simulink model "DMC_simulink_trial_1_MIMO"  (R2015a)
settings: Solver=ode45  StartTime=0.0  StopTime=900  RelTol=1e-3
values from neighbouring files (symbols this model uses):
  Fac = (inv(G'*G+lambda*eye(2*(M+1))))*(G')    [DMC_MIMO_DATA_Gen.m]    (also in DMC_SISO_DATA_Gen.m = (inv(G'*G+lambda*eye(M+1)))*(G'))
  temp_f = [temp_f_11 temp_f_12;temp_f_21 temp_f_22]    [DMC_MIMO_DATA_Gen.m]    (also in DMC_SISO_DATA_Gen.m = temp_g1 - temp_g2)
settings Model: Creator=Ronak  LastModifiedBy=Ronak

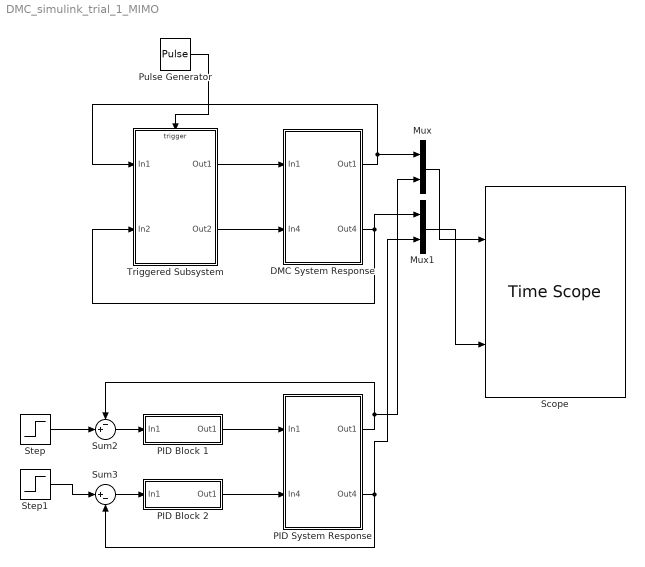
== system DMC_simulink_trial_1_MIMO ==
  DMC System Response : Subsystem
  Mux : Mux  Inputs=2
  Mux1 : Mux  Inputs=2
  PID Block 1 : Subsystem
  PID Block 2 : Subsystem
  PID System Response : Subsystem
  Pulse Generator : DiscretePulseGenerator  PulseType=Time based  Period=0.1  PulseWidth=5
  Scope : TimeScope  NumInputPorts=2
  Step : Step  SampleTime=0
  Step1 : Step  SampleTime=0
  Sum2 : Sum  Inputs=-+|
  Sum3 : Sum  Inputs=|+-
  Triggered Subsystem : Subsystem  TreatAsAtomicUnit=on
  wires:
  DMC System Response/1(Out1) -> Mux/1, Triggered Subsystem/1(In1)
  DMC System Response/2(Out4) -> Triggered Subsystem/2(In2), Mux1/1
  Pulse Generator/1 -> Triggered Subsystem/Trigger
  Triggered Subsystem/1(Out1) -> DMC System Response/1(In1)
  Triggered Subsystem/2(Out2) -> DMC System Response/2(In4)
  Mux/1 -> Scope/1
  Mux1/1 -> Scope/2
  PID Block 1/1(Out1) -> PID System Response/1(In1)
  PID Block 2/1(Out1) -> PID System Response/2(In4)
  Sum2/1 -> PID Block 1/1(In1)
  Sum3/1 -> PID Block 2/1(In1)
  Step/1 -> Sum2/2
  Step1/1 -> Sum3/1
  PID System Response/1(Out1) -> Mux/2, Sum2/1
  PID System Response/2(Out4) -> Sum3/2, Mux1/2

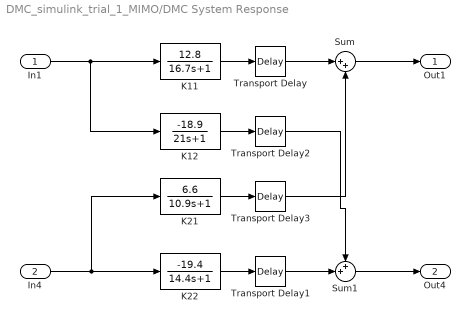
== system DMC_simulink_trial_1_MIMO/DMC System Response ==
  In1 : Inport
  In4 : Inport  Port=2
  K11 : TransferFcn  Numerator=[12.8]  Denominator=[16.7 1]
  K12 : TransferFcn  Numerator=[-18.9]  Denominator=[21 1]
  K21 : TransferFcn  Numerator=[6.6]  Denominator=[10.9 1]
  K22 : TransferFcn  Numerator=[-19.4]  Denominator=[14.4 1]
  Sum : Sum  Inputs=|++
  Sum1 : Sum  Inputs=++|
  Transport Delay : TransportDelay
  Transport Delay1 : TransportDelay  DelayTime=3
  Transport Delay2 : TransportDelay  DelayTime=3
  Transport Delay3 : TransportDelay  DelayTime=7
  Out1 : Outport
  Out4 : Outport  Port=2
  wires:
  In4/1 -> K21/1, K22/1
  K22/1 -> Transport Delay1/1
  In1/1 -> K12/1, K11/1
  Transport Delay1/1 -> Sum1/2
  K21/1 -> Transport Delay3/1
  K11/1 -> Transport Delay/1
  K12/1 -> Transport Delay2/1
  Sum1/1 -> Out4/1
  Sum/1 -> Out1/1
  Transport Delay/1 -> Sum/1
  Transport Delay2/1 -> Sum1/1
  Transport Delay3/1 -> Sum/2

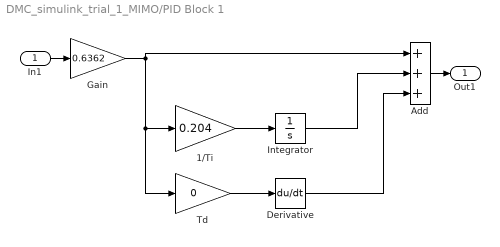
== system DMC_simulink_trial_1_MIMO/PID Block 1 ==
  In1 : Inport
  1/Ti : Gain  Gain=0.204
  Add : Sum  Inputs=+++
  Derivative : Derivative
  Gain : Gain  Gain=0.6362
  Integrator : Integrator
  Td : Gain  Gain=0
  Out1 : Outport
  wires:
  In1/1 -> Gain/1
  Add/1 -> Out1/1
  Gain/1 -> Add/1, Td/1, 1/Ti/1
  Integrator/1 -> Add/2
  Derivative/1 -> Add/3
  1/Ti/1 -> Integrator/1
  Td/1 -> Derivative/1

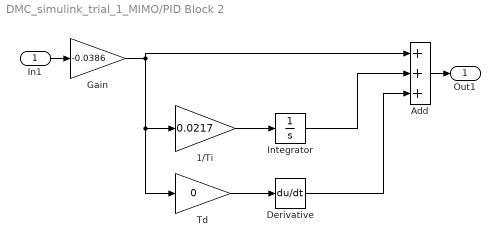
== system DMC_simulink_trial_1_MIMO/PID Block 2 ==
  In1 : Inport
  1/Ti : Gain  Gain=0.0217
  Add : Sum  Inputs=+++
  Derivative : Derivative
  Gain : Gain  Gain=-0.0386
  Integrator : Integrator
  Td : Gain  Gain=0
  Out1 : Outport
  wires:
  In1/1 -> Gain/1
  Add/1 -> Out1/1
  Gain/1 -> Add/1, Td/1, 1/Ti/1
  Integrator/1 -> Add/2
  Derivative/1 -> Add/3
  1/Ti/1 -> Integrator/1
  Td/1 -> Derivative/1

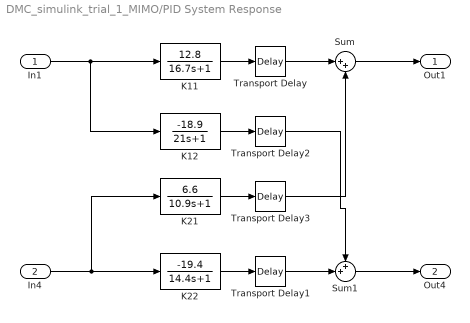
== system DMC_simulink_trial_1_MIMO/PID System Response ==
  In1 : Inport
  In4 : Inport  Port=2
  K11 : TransferFcn  Numerator=[12.8]  Denominator=[16.7 1]
  K12 : TransferFcn  Numerator=[-18.9]  Denominator=[21 1]
  K21 : TransferFcn  Numerator=[6.6]  Denominator=[10.9 1]
  K22 : TransferFcn  Numerator=[-19.4]  Denominator=[14.4 1]
  Sum : Sum  Inputs=|++
  Sum1 : Sum  Inputs=++|
  Transport Delay : TransportDelay
  Transport Delay1 : TransportDelay  DelayTime=3
  Transport Delay2 : TransportDelay  DelayTime=3
  Transport Delay3 : TransportDelay  DelayTime=7
  Out1 : Outport
  Out4 : Outport  Port=2
  wires:
  Transport Delay3/1 -> Sum/2
  Transport Delay2/1 -> Sum1/1
  Transport Delay/1 -> Sum/1
  Sum/1 -> Out1/1
  Sum1/1 -> Out4/1
  K12/1 -> Transport Delay2/1
  K11/1 -> Transport Delay/1
  K21/1 -> Transport Delay3/1
  Transport Delay1/1 -> Sum1/2
  In1/1 -> K11/1, K12/1
  K22/1 -> Transport Delay1/1
  In4/1 -> K22/1, K21/1

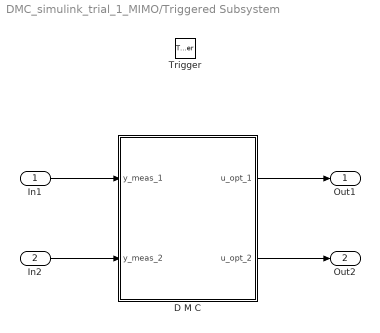
== system DMC_simulink_trial_1_MIMO/Triggered Subsystem ==
  In1 : Inport
  In2 : Inport  Port=2
  Trigger : TriggerPort
  D M C : MATLAB Function  TreatAsAtomicUnit=on
  Out1 : Outport
  Out2 : Outport  Port=2
  wires:
  In1/1 -> D M C/1(y_meas_1)
  D M C/1(u_opt_1) -> Out1/1
  D M C/2(u_opt_2) -> Out2/1
  In2/1 -> D M C/2(y_meas_2)

== matlab function DMC_simulink_trial_1_MIMO/Triggered Subsystem/D M C ==
  data: y_meas_1 input; y_meas_2 input; temp_f parameter; Fac parameter; u_opt_1 output; u_opt_2 output
function [u_opt_1,u_opt_2]    = fcn(y_meas_1,y_meas_2,temp_f,Fac)
%#codegen
coder.extrinsic('evalin', 'assignin')
r1 = y_meas_1;
r2 = y_meas_2;
y_sp_1 = 1;
y_sp_2 = 1;
alpha = 0.9;
u = zeros(2000,1);  % 2Nx1; past moves
u = evalin('base','u'); % Read value from workspace
u_old_1 = 0;
u_old_2 = 0;
u_old_1 = evalin('base','u_old_1'); 
u_old_2 = evalin('base','u_old_2'); 
ref_1 = zeros(1,900);       % 1,P
ref_2 = zeros(1,900);
for i =1:900    %1:P
    r1 = alpha*r1 + (1-alpha)*y_sp_1;
    r2 = alpha*r2 + (1-alpha)*y_sp_2;
    ref_1(i) = r1;
    ref_2(i) = r2;
end
ref = [ref_1';ref_2'];
f_1 = y_meas_1*ones(900,1);
f_2 = y_meas_2*ones(900,1);
y_meas = [f_1;f_2];
f = y_meas + temp_f*u; % Free Response
u_temp = Fac*(ref-f);
u_opt_1 = u_old_1 + u_temp(1);
u_opt_2 = u_old_2 + u_temp(601);
u = [u_temp(1);u(1:999);u_temp(601);u(1001:1999)];
assignin('base','u',u);
assignin('base','u_old_1',u_opt_1);
assignin('base','u_old_2',u_opt_2);
end
